simulink model "ThirdOrderCascadeSingleBitSC"  (R2023b)
settings: Solver=VariableStepDiscrete  StartTime=0.0  StopTime=(N-1)*Ts  RelTol=1e-3  EnableMultiTasking=on
undefined symbols (not defined in the file): Ain, ao1, ao2, avnl1, avnl2, avnl3, avnl4, Cint1, Cint2, cload, cnl1, cnl2, cpar1, cpar2, Cs11, Cs12, Cs21, Cs22, fin, gm1, gm2, innoise1, innoise2, io1, io2, osp, ron1, ron2, temp, Ts, vref
libraries: fesclib x3, quantrealib x2
settings Model: SimulationMode=accelerator  Creator=moreno  LastModifiedBy=pablo
settings SolverCC: AlgebraicLoopSolver=TrustRegion
settings DataIOCC: LimitDataPoints=on  SaveFormat=Array  ReturnWorkspaceOutputs=off  SignalLoggingName=sigsOut
settings OptimizationCC: BooleanDataType=off  ExpressionDepthLimit=2147483647  LifeSpan=inf
settings DebuggingCC: SaveWithParameterizedLinksMsg=none  UnderspecifiedInitializationDetection=Classic  MergeDetectMultiDrivingBlocksExec=none  SignalResolutionControl=TryResolveAllWithWarning  MultiTaskDSMMsg=warning  MultiTaskCondExecSysMsg=none  FcnCallInpInsideContextMsg=warning  UnconnectedInputMsg=warning  UnconnectedOutputMsg=warning  StateNameClashWarn=warning  SFUnexpectedBacktrackingDiag=warning  SFNoUnconditionalDefaultTransitionDiag=warning  SFExecutionAtInitializationDiag=none  ArithmeticOperatorsInVariantConditions=warning
settings HardwareCC: ProdBitPerPointer=32  ProdBitPerSizeT=32  ProdBitPerPtrDiffT=32  ProdLargestAtomicFloat=None  ProdIntDivRoundTo=Undefined  ProdEndianess=Unspecified  ProdWordSize=32  ProdHWDeviceType=32-bit Generic  TargetUnknown=on
settings ModelReferenceCC: EnableRefExpFcnMdlSchedulingChecks=on  PropagateSignalLabelsOutOfModel=off
settings SFSimCC: SimUseLocalCustomCode=off  CustomCodeUndefinedFunction=UseInterfaceOnly
settings RTWCC: RTWUseLocalCustomCode=off  DLArmComputeVersion=19.05
settings CodeAppCC: StateflowObjectComments=on
settings GRTTargetCC: TargetLangStandard=C89/C90 (ANSI)  CombineOutputUpdateFcns=off  GRTInterface=on
settings ConfigComp: CovMetricSettings=dw  CovSaveCumulativeToWorkspaceVar=on  CovSaveSingleToWorkspaceVar=on  CovExternalEMLEnable=off

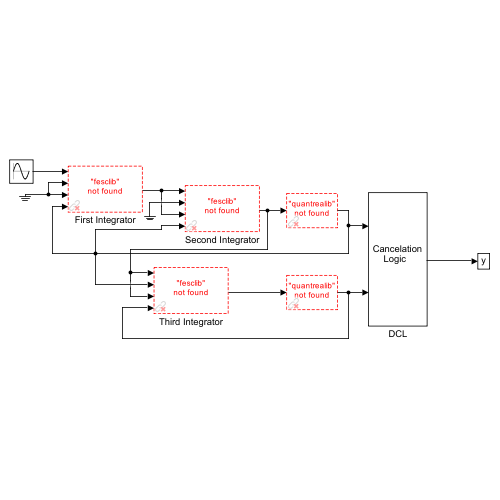
[thumbnail: Simulink's stored preview of the top-level diagram]
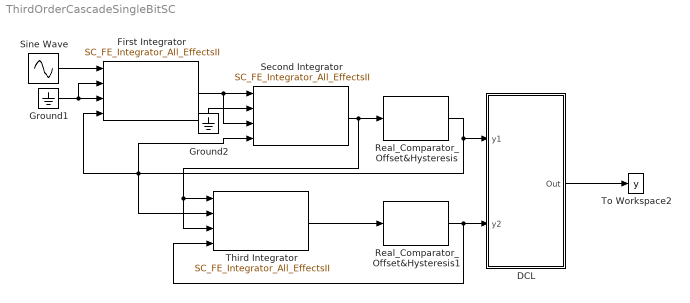
== system ThirdOrderCascadeSingleBitSC ==
  DCL : Subsystem
      mask Display: disp(strvcat('Cancelation','  Logic'))
  First Integrator : fesclib/SC_FE_Integrator_All_EffectsII  c=[Cint1,Cs11,Cs21,cnl1,cnl2]  var=[0,innoise1,temp,ron1]  ops=[osp,-osp]  ao=[ao1,gm1,io1]  avnl=[avnl1,avnl2,avnl3,avnl4]  cp=[cpar1,cpar2,cload]  phi=phi1  ts=Ts  settlingon=on  setin=on  idown=a  idnext=b
      link override C11: Value=6e-12
      link override C12: Value=6e-12
      link override From: GotoTag=b
      link override Goto: GotoTag=a
  Ground1 : Ground
  Ground2 : Ground
  Real_Comparator_Offset&Hysteresis : quantrealib/Real_Comparator_Offset&Hysteresis  Vhigh=vref  Vlow=-vref  OFFSET_PARAM=0  FLAG_PARAM=Without Hysteresys  H_PARAM=hys  phi=phi1  ts=Ts  qid=quant1
      link override Goto: GotoTag=quant1
  Real_Comparator_Offset&Hysteresis1 : quantrealib/Real_Comparator_Offset&Hysteresis  Vhigh=vref  Vlow=-vref  OFFSET_PARAM=0  FLAG_PARAM=Without Hysteresys  H_PARAM=hys  phi=phi1  ts=Ts  qid=quant2
      link override Goto: GotoTag=quant2
  Second Integrator : fesclib/SC_FE_Integrator_All_EffectsII  c=[Cint2,Cs12,Cs22,cnl1,cnl2]  var=[0,innoise2,temp,ron2]  ops=[osp,-osp]  ao=[ao2,gm2,io2]  avnl=[avnl1,avnl2,avnl3,avnl4]  cp=[cpar1,cpar2,cload]  phi=phi1  ts=Ts  settlingon=on  setin=on  idown=b  idnext=c
      link override C11: Value=1.5e-12
      link override C12: Value=1.5e-12
      link override From: GotoTag=c
      link override Goto: GotoTag=b
  Sine Wave : Sin  Amplitude=10^(Ain/20)  Frequency=2*pi*fin  SampleTime=0
  Third Integrator : fesclib/SC_FE_Integrator_All_EffectsII  c=[Cint2,Cs12,Cs22,cnl1,cnl2]  var=[0,innoise2,temp,ron2]  ops=[osp,-osp]  ao=[ao2,gm2,io2]  avnl=[avnl1,avnl2,avnl3,avnl4]  cp=[cpar1,cpar2,cload]  phi=phi1  ts=Ts  settlingon=on  setin=off  idown=c  idnext=c
      link override C11: Value=1.5e-12
      link override C12: Value=1.5e-12
      link override From: GotoTag=c
      link override Goto: GotoTag=c
  To Workspace2 : ToWorkspace  VariableName=y  SampleTime=Ts
      settings: MaxDataPoints=N
  wires:
  Sine Wave/1 -> First Integrator/1
  First Integrator/1 -> Second Integrator/3, Second Integrator/1
  Second Integrator/1 -> Real_Comparator_Offset&Hysteresis/1, Third Integrator/3, Third Integrator/1
  Real_Comparator_Offset&Hysteresis/1 -> DCL/1(y1), Third Integrator/2, First Integrator/4, Second Integrator/4
  Third Integrator/1 -> Real_Comparator_Offset&Hysteresis1/1
  Real_Comparator_Offset&Hysteresis1/1 -> DCL/2(y2), Third Integrator/4
  Ground2/1 -> Second Integrator/2
  DCL/1(Out) -> To Workspace2/1
  Ground1/1 -> First Integrator/3, First Integrator/2

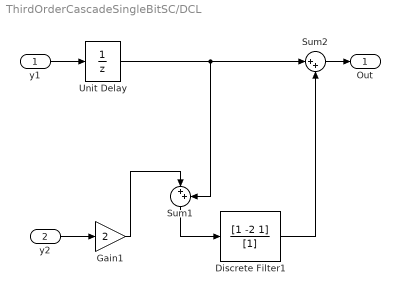
== system ThirdOrderCascadeSingleBitSC/DCL ==
  y1 : Inport
  y2 : Inport  Port=2
  Discrete Filter1 : DiscreteFilter  Numerator=[1 -2 1]  Denominator=[1]  SampleTime=Ts
  Gain1 : Gain  Gain=2  SaturateOnIntegerOverflow=on  OutDataTypeStr=Inherit: Same as input  ParamDataTypeStr=Inherit: Same as input
  Sum1 : Sum  Inputs=|++  InputSameDT=on  SaturateOnIntegerOverflow=on  OutDataTypeStr=Inherit: Same as first input
  Sum2 : Sum  Inputs=|++  InputSameDT=on  SaturateOnIntegerOverflow=on  OutDataTypeStr=Inherit: Same as first input
  Unit Delay : UnitDelay  SampleTime=Ts  HasFrameUpgradeWarning=on
  Out : Outport
  wires:
  Unit Delay/1 -> Sum2/1, Sum1/2
  Discrete Filter1/1 -> Sum2/2
  Gain1/1 -> Sum1/1
  Sum1/1 -> Discrete Filter1/1
  y1/1 -> Unit Delay/1
  y2/1 -> Gain1/1
  Sum2/1 -> Out/1
